simulink model "sim_identification"  (R2024b)
settings: Solver=ode4  StartTime=0.0  StopTime=T_SIMULATION  FixedStep=T_s  RelTol=1e-3
values from neighbouring files (symbols this model uses):
  d = d_nominal    (= 0.165)    [id_LEO.m]    (also in init_localization.m; init_localization_template.m; script_init_localization.m)
  PHI_INIT = [0 0]    [data_for_identification.mat]    (also in id_LEO.m = [0;0]; id_template.m = [0;0]; init_localization.m = [0;0]; init_localization_template.m = [0;0])
  Q_INIT = [0 0 0.463647609001]    [data_for_identification.mat]    (also in id_LEO.m = q(:,1); id_template.m = [0;0;atan(0.5)]; init_localization.m = [0;0;0]; script_init_localization.m = q(:,1))
  r = r_nominal    (= 0.03)    [id_LEO.m]    (also in init_localization.m; init_localization_template.m; script_init_localization.m)
  T_s = Ts_values(i)    [EX_opt_1.m]    (also in EX_opt_2.m; data_for_identification.mat = 0.04; id_LEO.m = 0.04; id_template.m = 0.04)
undefined symbols (not defined in the file or in its folder): Ts
settings Model: Creator=llp  LastModifiedBy=loren

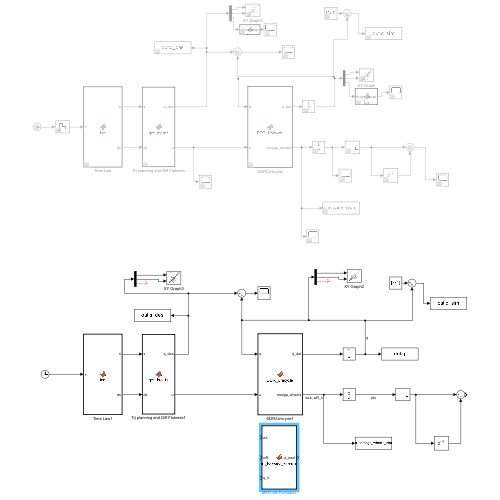
[thumbnail: Simulink's stored preview of the top-level diagram]
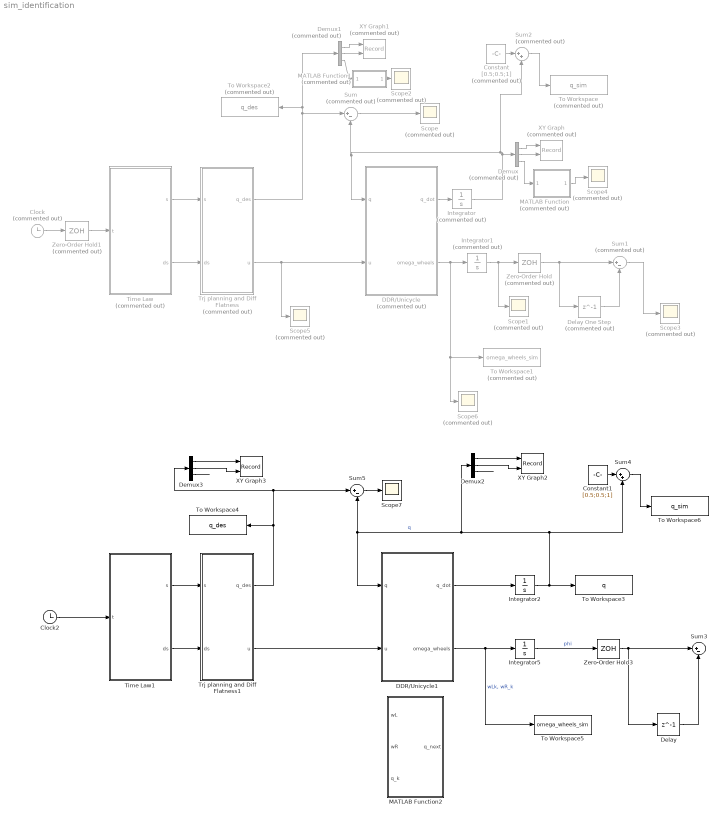
== system sim_identification ==
  Clock : Clock  Commented=on
  Clock2 : Clock
  Constant : Constant  Commented=on  Value=[0.5;0.5;1]
  Constant1 : Constant  Value=[0.5;0.5;1]
  DDR/Unicycle : MATLAB Function  Commented=on  TreatAsAtomicUnit=on
  DDR/Unicycle1 : MATLAB Function  TreatAsAtomicUnit=on
  Delay : Delay  DelayLength=1  InitialCondition=[0;0]  SampleTime=T_s
  Delay One Step : Delay  Commented=on  DelayLength=1  SampleTime=T_s
  Demux : Demux  Commented=on  Outputs=3
  Demux1 : Demux  Commented=on  Outputs=3
  Demux2 : Demux  Outputs=3
  Demux3 : Demux  Outputs=3
  Integrator : Integrator  Commented=on  InitialCondition=Q_INIT
  Integrator1 : Integrator  Commented=on  InitialCondition=PHI_INIT
  Integrator2 : Integrator  InitialCondition=Q_INIT
  Integrator5 : Integrator  InitialCondition=PHI_INIT
  MATLAB Function : MATLAB Function  Commented=on  TreatAsAtomicUnit=on
  MATLAB Function1 : MATLAB Function  Commented=on  TreatAsAtomicUnit=on
  MATLAB Function2 : MATLAB Function  TreatAsAtomicUnit=on
  Scope{,1..6} (7 alike) : Scope  Commented=on
  Scope7 : Scope
  Sum : Sum  Commented=on  Inputs=|+-
  Sum1 : Sum  Commented=on  Inputs=|+-
  Sum2 : Sum  Commented=on  Inputs=|++
  Sum3 : Sum  Inputs=|+-
  Sum4 : Sum  Inputs=|++
  Sum5 : Sum  Inputs=|+-
  Time Law : MATLAB Function  Commented=on  TreatAsAtomicUnit=on
  Time Law1 : MATLAB Function  TreatAsAtomicUnit=on
  To Workspace : ToWorkspace  Commented=on  VariableName=q_sim  SaveFormat=Structure With Time  SampleTime=-1
  To Workspace1 : ToWorkspace  Commented=on  VariableName=omega_wheels_sim  SaveFormat=Structure With Time  SampleTime=-1
  To Workspace2 : ToWorkspace  Commented=on  VariableName=q_des  SaveFormat=Structure With Time  SampleTime=-1
  To Workspace3 : ToWorkspace  VariableName=q  SaveFormat=Structure With Time  SampleTime=-1
  To Workspace4 : ToWorkspace  VariableName=q_des  SaveFormat=Structure With Time  SampleTime=-1
  To Workspace5 : ToWorkspace  VariableName=omega_wheels_sim  SaveFormat=Structure With Time  SampleTime=-1
  To Workspace6 : ToWorkspace  VariableName=q_sim  SaveFormat=Structure With Time  SampleTime=-1
  Trj planning and Diff Flatness : MATLAB Function  Commented=on  TreatAsAtomicUnit=on
  Trj planning and Diff Flatness1 : MATLAB Function  TreatAsAtomicUnit=on
  XY Graph : Record  Commented=on  FileSettingsInternal="{\"entries\":[{\"content\":{\"excelSettings\":{\"content\":{},\"type\":\"Streamout.ExcelSettings\"}},\"type\":\"Streamout.FileSettingStorage\",\"uuid\":\"\"}],\"packageUris\":[\"http:\\/\\/schema.mathworks.com\\/mf0\\/streamout_blocks\\/R2020a\"],\"version\":\"1.0\"}"  Layout=[1 1]  SignalsInternal="{\"entries\":[{\"content\":{},\"type\":\"RecordBlkView.InputSignals\",\"uuid\":\"\"}],\"packageUris\":[\"http:\\/\\/schema.mathworks.com\\/mf0\\/streamout_blocks\\/R2020a\"],\"version\":\"1.0\"}"  VisualizationBindings="{\"xyplotplugin\":{\"info\":[{\"series\":[],\"subplotID\":1}]}}"  CompatibilityTag=XY
  XY Graph1 : Record  Commented=on  FileSettingsInternal="{\"entries\":[{\"content\":{\"excelSettings\":{\"content\":{},\"type\":\"Streamout.ExcelSettings\"}},\"type\":\"Streamout.FileSettingStorage\",\"uuid\":\"\"}],\"packageUris\":[\"http:\\/\\/schema.mathworks.com\\/mf0\\/streamout_blocks\\/R2020a\"],\"version\":\"1.0\"}"  Layout=[1 1]  SignalsInternal="{\"entries\":[{\"content\":{},\"type\":\"RecordBlkView.InputSignals\",\"uuid\":\"\"}],\"packageUris\":[\"http:\\/\\/schema.mathworks.com\\/mf0\\/streamout_blocks\\/R2020a\"],\"version\":\"1.0\"}"  VisualizationBindings="{\"xyplotplugin\":{\"info\":[{\"series\":[],\"subplotID\":1}]}}"  CompatibilityTag=XY
  XY Graph2 : Record  FileSettingsInternal="{\"entries\":[{\"content\":{\"excelSettings\":{\"content\":{},\"type\":\"Streamout.ExcelSettings\"}},\"type\":\"Streamout.FileSettingStorage\",\"uuid\":\"\"}],\"packageUris\":[\"http:\\/\\/schema.mathworks.com\\/mf0\\/streamout_blocks\\/R2020a\"],\"version\":\"1.0\"}"  Layout=[1 1]  SignalsInternal="{\"entries\":[{\"content\":{\"signals\":[{\"content\":{\"blockPath\":[],\"dimensions\":[1,1],\"domain\":\"\",\"lineColor\":\"#a2142f\",\"plots\":[ 1 ],\"port\":1,\"sid\":[\"\"],\"signalID\":1,\"signalName\":\"Demux2:1\"},\"type\":\"RecordBlkView.Signal\",\"uuid\":\"\"},{\"content\":{\"blockPath\":[],\"dimensions\":[1,1],\"domain\":\"\",\"lineColor\":\"#139fff\",\"plots\":[ 1 ],\"port\":2,\"sid\":[\"\"],\"signalID\":2,\"signalName\":\"Demux2:2\"},\"type\":\"RecordBlkView.Signal\",\"uuid\":\"\"}]},\"type\":\"RecordBlkView.InputSignals\",\"uuid\":\"\"}],\"packageUris\":[\"http:\\/\\/schema.mathworks.com\\/mf0\\/streamout_blocks\\/R2020a\"],\"version\":\"1.0\"}"  VisualizationBindings="{\"xyplotplugin\":{\"info\":[{\"series\":[{\"bindingParametersList\":[{\"parameter\":\"X-Axis\",\"signalID\":1,\"signalName\":\"Demux2:1\"},{\"parameter\":\"Y-Axis\",\"signalID\":2,\"signalName\":\"Demux2:2\"}],\"seriesID\":0}],\"subplotID\":1}]}}"  CompatibilityTag=XY
  XY Graph3 : Record  FileSettingsInternal="{\"entries\":[{\"content\":{\"excelSettings\":{\"content\":{},\"type\":\"Streamout.ExcelSettings\"}},\"type\":\"Streamout.FileSettingStorage\",\"uuid\":\"\"}],\"packageUris\":[\"http:\\/\\/schema.mathworks.com\\/mf0\\/streamout_blocks\\/R2020a\"],\"version\":\"1.0\"}"  Layout=[1 1]  SignalsInternal="{\"entries\":[{\"content\":{\"signals\":[{\"content\":{\"blockPath\":[],\"dimensions\":[1,1],\"domain\":\"\",\"lineColor\":\"#a2142f\",\"plots\":[ 1 ],\"port\":1,\"sid\":[\"\"],\"signalID\":1,\"signalName\":\"Demux3:1\"},\"type\":\"RecordBlkView.Signal\",\"uuid\":\"\"},{\"content\":{\"blockPath\":[],\"dimensions\":[1,1],\"domain\":\"\",\"lineColor\":\"#139fff\",\"plots\":[ 1 ],\"port\":2,\"sid\":[\"\"],\"signalID\":2,\"signalName\":\"Demux3:2\"},\"type\":\"RecordBlkView.Signal\",\"uuid\":\"\"}]},\"type\":\"RecordBlkView.InputSignals\",\"uuid\":\"\"}],\"packageUris\":[\"http:\\/\\/schema.mathworks.com\\/mf0\\/streamout_blocks\\/R2020a\"],\"version\":\"1.0\"}"  VisualizationBindings="{\"xyplotplugin\":{\"info\":[{\"series\":[{\"bindingParametersList\":[{\"parameter\":\"X-Axis\",\"signalID\":1,\"signalName\":\"Demux3:1\"},{\"parameter\":\"Y-Axis\",\"signalID\":2,\"signalName\":\"Demux3:2\"}],\"seriesID\":0}],\"subplotID\":1}]}}"  CompatibilityTag=XY
  Zero-Order Hold : ZeroOrderHold  Commented=on  SampleTime=T_s
  Zero-Order Hold1 : ZeroOrderHold  Commented=on  SampleTime=T_s
  Zero-Order Hold3 : ZeroOrderHold  SampleTime=T_s
  wires:
  Clock/1 -> Zero-Order Hold1/1
  Time Law/1(s) -> Trj planning and Diff Flatness/1(s)
  Time Law/2(ds) -> Trj planning and Diff Flatness/2(ds)
  DDR/Unicycle/1(q_dot) -> Integrator/1
  Trj planning and Diff Flatness/2(u) -> Scope5/1, DDR/Unicycle/2(u)
  Integrator/1 -> Demux/1, Sum/2, DDR/Unicycle/1(q), Sum2/2
  Trj planning and Diff Flatness/1(q_des) -> Demux1/1, To Workspace2/1, Sum/1
  Sum/1 -> Scope/1
  DDR/Unicycle/2(omega_wheels) -> Scope6/1, To Workspace1/1, Integrator1/1
  Integrator1/1 -> Zero-Order Hold/1, Scope1/1
  Demux/1 -> XY Graph/1
  Demux/2 -> XY Graph/2
  Demux/3 -> MATLAB Function/1(theta)
  Demux1/2 -> XY Graph1/2
  Demux1/3 -> MATLAB Function1/1(theta)
  Demux1/1 -> XY Graph1/1
  MATLAB Function/1(wrap) -> Scope4/1
  MATLAB Function1/1(wrap) -> Scope2/1
  Zero-Order Hold/1 -> Delay One Step/1, Sum1/1
  Delay One Step/1 -> Sum1/2
  Sum1/1 -> Scope3/1
  Zero-Order Hold1/1 -> Time Law/1(t)
  Constant/1 -> Sum2/1
  Sum2/1 -> To Workspace/1
  Demux3/3 -> ?
  Demux2/3 -> ?
  Demux2/2 -> XY Graph2/2
  Demux2/1 -> XY Graph2/1
  Delay/1 -> Sum3/2
  Demux3/1 -> XY Graph3/1
  Zero-Order Hold3/1 -> Sum3/1, Delay/1
  Integrator5/1 -> Zero-Order Hold3/1  "phi"
  Integrator2/1 -> Sum4/2, DDR/Unicycle1/1(q), Sum5/2, Demux2/1, To Workspace3/1  "q"
  Time Law1/2(ds) -> Trj planning and Diff Flatness1/2(ds)
  Sum5/1 -> Scope7/1
  DDR/Unicycle1/1(q_dot) -> Integrator2/1
  Time Law1/1(s) -> Trj planning and Diff Flatness1/1(s)
  DDR/Unicycle1/2(omega_wheels) -> Integrator5/1, To Workspace5/1  "wLk, wR_k"
  Demux3/2 -> XY Graph3/2
  Trj planning and Diff Flatness1/1(q_des) -> To Workspace4/1, Sum5/1, Demux3/1
  Clock2/1 -> Time Law1/1(t)
  Sum4/1 -> To Workspace6/1
  Constant1/1 -> Sum4/1
  Trj planning and Diff Flatness1/2(u) -> DDR/Unicycle1/2(u)

== matlab function sim_identification/Time Law ==
  data: t input; s output; ds output
function [s, ds] = fcn(t)
    
    Ta = 0.5;
    Tc = 9; 
        
    vc = 1/(Ta+Tc);
    a = vc/Ta;
   
    if t < Ta
        s_dot = a*t;
        s = 0.5*a*t^2;
    
    elseif t < (Ta+Tc)
        s_dot = vc;
        s = 0.5*a*Ta^2 + vc*(t - Ta);
    
    elseif t < (2*Ta+Tc)
        s_dot = vc - a*(t - Ta - Tc);
        s = 0.5*a*Ta^2 + vc*Tc + vc*(t - Ta - Tc) ...
            - 0.5*a*(t - Ta - Tc)^2;
    else
        s_dot = 0;
        s = 1;
    end

    ds = s_dot;
    
end

== matlab function sim_identification/DDR//Unicycle ==
  data: q input; u input; q_dot output; omega_wheels output; d parameter; r parameter
function [q_dot, omega_wheels] = DDR_Unicycle(q, u, d, r)

    % extract variables
    v = u(1);
    omega = u(2);

    q_dot= zeros(3,1);
    
    q_dot(1) = v*cos(q(3));
    q_dot(2) = v*sin(q(3));
    q_dot(3) = omega;

    
    wL = v/r - d/(2*r) * omega;
    wR = v/r + d/(2*r) * omega;

    omega_wheels = [wL; wR];

end

== matlab function sim_identification/Trj planning and Diff Flatness ==
  data: q_des output; s input; u output; ds input
function [q_des, u] = get_inputs(s, ds)

R = 0.4;
omega = 2*pi;

x = R*sin(2*omega*s);
y = R*sin(omega*s);

dx_ds = 2*omega*R*cos(2*omega*s);
dy_ds = omega*R*cos(omega*s);

ddx_ds2 = -4*omega^2*R*sin(2*omega*s);
ddy_ds2 = -omega^2*R*sin(omega*s);



theta = atan2(dy_ds, dx_ds);

q_des = [x; y; theta];

v = ds* sqrt(dx_ds^2 + dy_ds^2);

omega_input = ds* (dx_ds*ddy_ds2 - dy_ds*ddx_ds2) / (dx_ds^2 + dy_ds^2+10^-3);

u = [v; omega_input];

end

== matlab function sim_identification/MATLAB Function ==
  data: theta input; wrap output
function wrap = fcn(theta)

wrap = mod(theta+pi,2*pi)-pi ;

== matlab function sim_identification/MATLAB Function1 ==
  data: theta input; wrap output
function wrap = fcn(theta)

wrap = mod(theta+pi,2*pi)-pi ;

== matlab function sim_identification/DDR//Unicycle1 ==
  data: q input; u input; q_dot output; omega_wheels output; d parameter; r parameter
function [q_dot, omega_wheels] = DDR_Unicycle(q, u, d, r)

    % extract variables
    v = u(1);
    omega = u(2);

    q_dot= zeros(3,1);
    
    q_dot(1) = v*cos(q(3));
    q_dot(2) = v*sin(q(3));
    q_dot(3) = omega;

    
    wL = v/r - d/(2*r) * omega;
    wR = v/r + d/(2*r) * omega;

    omega_wheels = [wL; wR];

end

== matlab function sim_identification/Time Law1 ==
  data: t input; s output; ds output
function [s, ds] = fcn(t)
    
    Ta = 0.5;
    Tc = 9; 
        
    vc = 1/(Ta+Tc);
    a = vc/Ta;
   
    if t < Ta
        s_dot = a*t;
        s = 0.5*a*t^2;
    
    elseif t < (Ta+Tc)
        s_dot = vc;
        s = 0.5*a*Ta^2 + vc*(t - Ta);
    
    elseif t < (2*Ta+Tc)
        s_dot = vc - a*(t - Ta - Tc);
        s = 0.5*a*Ta^2 + vc*Tc + vc*(t - Ta - Tc) ...
            - 0.5*a*(t - Ta - Tc)^2;
    else
        s_dot = 0;
        s = 1;
    end

    ds = s_dot;
    
end

== matlab function sim_identification/Trj planning and Diff Flatness1 ==
  data: q_des output; s input; u output; ds input
function [q_des, u] = get_inputs(s, ds)

    R = 0.4;
    w = 2*pi;

    % function [x_s, y_s, x_s_dot, y_s_dot, x_s_ddot, y_s_ddot] = gen_eight_shape_trajectory(R, w, s)
   
    x_s = R*sin(2*w*s);
    y_s = R*sin(w*s);
    
    % computes derivatives analytically

    x_s_dot = 2*R*w*cos(2*w*s);
    y_s_dot = R*w*cos(w*s);
    
    x_s_ddot = -4*R*w^2*sin(2*w*s);
    y_s_ddot = -R*w^2*sin(w*s);


    % function [q, u] = flat_to_kinematic_cartesian(x, y, x_dot, y_dot, x_ddot, y_ddot)

    theta = atan2(y_s_dot, x_s_dot);
    
    q_des = [x_s; y_s; theta];
   
    v_tilde = sqrt(x_s_dot^2 + y_s_dot^2);
    omega_tilde = (x_s_dot * y_s_ddot - y_s_dot * x_s_ddot) / (x_s_dot^2 + y_s_dot^2);
    
    % Convert into real Inputs
    v = v_tilde * ds;
    omega = omega_tilde * ds;
    
    u = [v; omega];
end

== matlab function sim_identification/MATLAB Function2 ==
  data: wL input; q_next output; wR input; q_k input; r parameter; d parameter; Ts parameter
function q_next = euler_forward_kinematics(wL, wR, q_k, r, d, Ts)
    % Reconstruct kinematic inputs from wheels
    v = (r / 2) * (wR + wL);
    w = (r / d) * (wR - wL);
    
    % Euler integration to perfectly match get_phi_reg assumption
    x_next = q_k(1) + v * Ts * cos(q_k(3));
    y_next = q_k(2) + v * Ts * sin(q_k(3));
    theta_next = q_k(3) + w * Ts;
    
    q_next = [x_next; y_next; theta_next];
end
